simulink model "modelNew"  (R2015a)
settings: Solver=ode45  StartTime=0.0  StopTime=10  RelTol=1e-3
values from neighbouring files (symbols this model uses):
  Aref = [0,1,0 ... (first row only)    [script.m]
  B = [0; gamma/(R*M);0]    [script.m]
  Bref = [0;0;a0]    [script.m]
  GammaX = theta(1)*eye(3)    [script.m]
  P = lyap(Aref',theta(2)*eye(3))    [script.m]
settings Model: Creator=user  LastModifiedBy=user

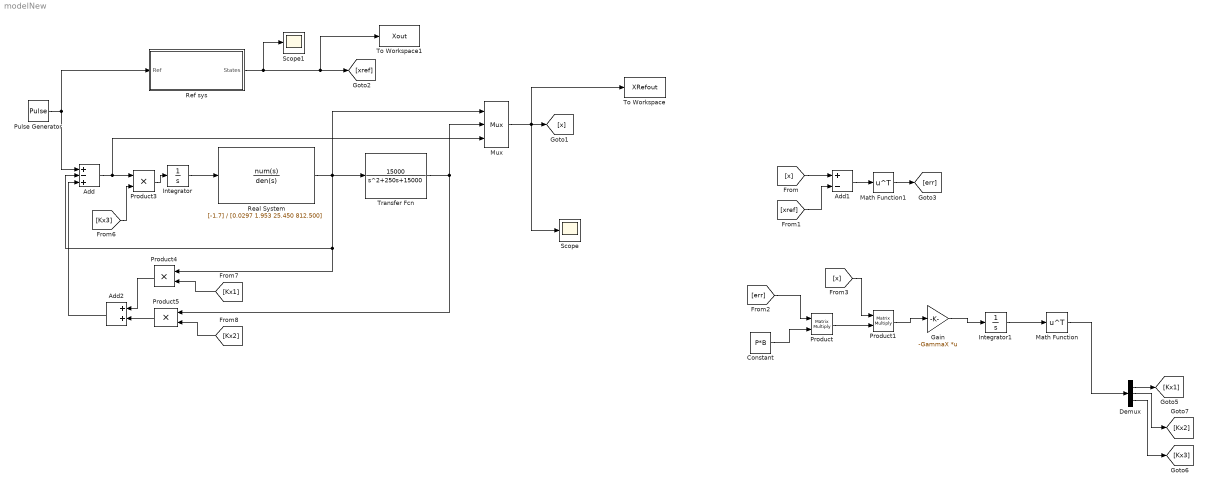
== system modelNew ==
  Add : Sum  Inputs=+-+
  Add1 : Sum  Inputs=+-
  Add2 : Sum
  Constant : Constant  Value=P*B
  Demux : Demux  Outputs=3
  Gain : Gain  Gain=-GammaX  Multiplication=Matrix(K*u)
  Integrator : Integrator
  Integrator1 : Integrator
  Math Function : Math  Operator=transpose  SaturateOnIntegerOverflow=on
  Math Function1 : Math  Operator=transpose  SaturateOnIntegerOverflow=on
  Mux : Mux  Inputs=3
  Product : Product  Multiplication=Matrix(*)
  Product1 : Product  Multiplication=Matrix(*)
  Product3 : Product
  Product4 : Product
  Product5 : Product
  Pulse Generator : DiscretePulseGenerator  PulseType=Time based  Period=10  PulseWidth=50
  Real System : TransferFcn  Numerator=[-1.7]  Denominator=[0.0297 1.953 25.450 812.500]
  Ref sys : Subsystem
  Scope : Scope
  Scope1 : Scope
      settings: YMin=0  YMax=8.5
  To Workspace : ToWorkspace  VariableName=XRefout  SaveFormat=Timeseries  SampleTime=-1
  To Workspace1 : ToWorkspace  VariableName=Xout  SaveFormat=Timeseries  SampleTime=-1
  Transfer Fcn : TransferFcn  Numerator=15000  Denominator=[1 250 15000]
  wires:
  Pulse Generator/1 -> Ref sys/1(Ref), Add/1
  Integrator/1 -> Real System/1
  Real System/1 -> Mux/1, Add/2, Product4/1, Transfer Fcn/1
  Transfer Fcn/1 -> Mux/2, Product5/1
  Mux/1 -> To Workspace/1, Scope/1, [x]
  Ref sys/1(States) -> Scope1/1, To Workspace1/1, [xref]
  [x] -> Add1/1
  [xref] -> Add1/2
  [err] -> Product/1
  Constant/1 -> Product/2
  Product/1 -> Product1/2
  [x] -> Product1/1
  Product1/1 -> Gain/1
  Gain/1 -> Integrator1/1
  Integrator1/1 -> Math Function/1
  Math Function/1 -> Demux/1
  Add1/1 -> Math Function1/1
  Math Function1/1 -> [err]
  Add/1 -> Mux/3, Product3/1
  Product3/1 -> Integrator/1
  Demux/1 -> [Kx1]
  Demux/3 -> [Kx3]
  Demux/2 -> [Kx2]
  [Kx3] -> Product3/2
  [Kx1] -> Product4/2
  [Kx2] -> Product5/2
  Product4/1 -> Add2/1
  Product5/1 -> Add2/2
  Add2/1 -> Add/3

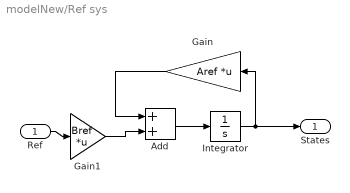
== system modelNew/Ref sys ==
  Ref : Inport
  Add : Sum
  Gain : Gain  Gain=Aref  Multiplication=Matrix(K*u)
  Gain1 : Gain  Gain=Bref  Multiplication=Matrix(K*u)
  Integrator : Integrator
  States : Outport
  wires:
  Gain/1 -> Add/1
  Gain1/1 -> Add/2
  Add/1 -> Integrator/1
  Ref/1 -> Gain1/1
  Integrator/1 -> States/1, Gain/1
